simulink model "byte8ram"  (R2019b)
settings: Solver=VariableStepAuto  StartTime=0.0  StopTime=10.0  RelTol=1e-3
libraries: simulink_extras x64
settings Model: Creator=kishan  LastModifiedBy=kishan

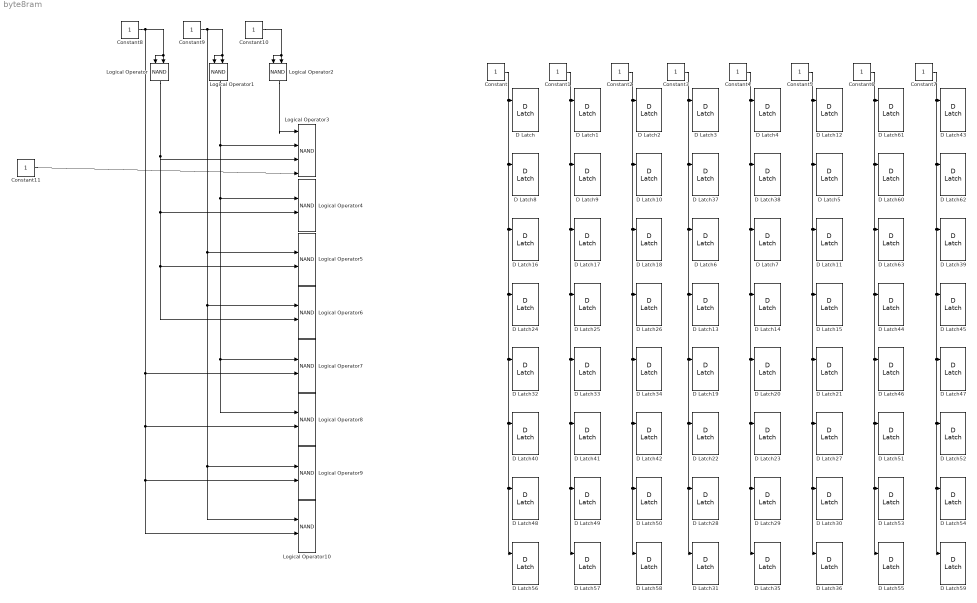
== system byte8ram ==
  Constant{,1..11} (12 alike) : Constant
  D Latch{,1..63} (64 alike) : simulink_extras/Flip Flops/D Latch
      settings: SourceProductName=Simulink  SourceProductBaseCode=SL
  Logical Operator : Logic  Operator=NAND  AllPortsSameDT=off  OutDataTypeStr=boolean
  Logical Operator1 : Logic  Operator=NAND  AllPortsSameDT=off  OutDataTypeStr=boolean
  Logical Operator{3..10} (8 alike) : Logic  Operator=NAND  Inputs=4  AllPortsSameDT=off  OutDataTypeStr=boolean
  Logical Operator2 : Logic  Operator=NAND  AllPortsSameDT=off  OutDataTypeStr=boolean
  wires:
  Constant/1 -> D Latch56/1, D Latch48/1, D Latch40/1, D Latch32/1, D Latch24/1, D Latch16/1, D Latch8/1, D Latch/1
  Constant1/1 -> D Latch57/1, D Latch49/1, D Latch41/1, D Latch33/1, D Latch25/1, D Latch17/1, D Latch9/1, D Latch1/1
  Constant2/1 -> D Latch58/1, D Latch50/1, D Latch42/1, D Latch34/1, D Latch26/1, D Latch18/1, D Latch10/1, D Latch2/1
  Constant5/1 -> D Latch36/1, D Latch30/1, D Latch27/1, D Latch21/1, D Latch15/1, D Latch11/1, D Latch5/1, D Latch12/1
  Constant3/1 -> D Latch31/1, D Latch28/1, D Latch22/1, D Latch19/1, D Latch13/1, D Latch6/1, D Latch37/1, D Latch3/1
  Constant4/1 -> D Latch35/1, D Latch29/1, D Latch23/1, D Latch20/1, D Latch14/1, D Latch7/1, D Latch38/1, D Latch4/1
  Constant7/1 -> D Latch59/1, D Latch54/1, D Latch52/1, D Latch47/1, D Latch45/1, D Latch39/1, D Latch62/1, D Latch43/1
  Constant6/1 -> D Latch55/1, D Latch53/1, D Latch51/1, D Latch46/1, D Latch44/1, D Latch63/1, D Latch60/1, D Latch61/1
  Constant8/1 -> Logical Operator10/3, Logical Operator9/3, Logical Operator8/3, Logical Operator7/3, Logical Operator/1, Logical Operator/2
  Constant9/1 -> Logical Operator10/2, Logical Operator9/2, Logical Operator6/2, Logical Operator5/2, Logical Operator1/1, Logical Operator1/2
  Constant10/1 -> Logical Operator2/1, Logical Operator2/2
  Logical Operator2/1 -> Logical Operator3/1
  Logical Operator1/1 -> Logical Operator8/2, Logical Operator7/2, Logical Operator4/2, Logical Operator3/2
  Logical Operator/1 -> Logical Operator6/3, Logical Operator5/3, Logical Operator4/3, Logical Operator3/3
  Constant11/1 -> Logical Operator3/4
